simulink model "untitled"  (R2017a)
settings: Solver=FixedStepAuto  StartTime=0.0  StopTime=inf  RelTol=1e-3
settings Model: Creator=teobaiguera  LastModifiedBy=teobaiguera

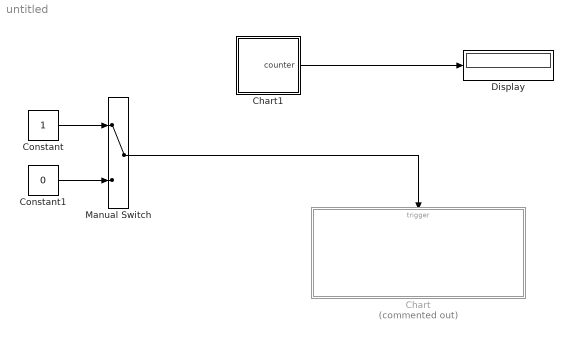
== system untitled ==
  Chart : Stateflow chart  Commented=on  TreatAsAtomicUnit=on
  Chart1 : Stateflow chart  TreatAsAtomicUnit=on
  Constant : Constant
  Constant1 : Constant  Value=0
  Display : Display
  Manual Switch : ManualSwitch
  wires:
  Constant/1 -> Manual Switch/1
  Constant1/1 -> Manual Switch/2
  Manual Switch/1 -> Chart/Trigger
  Chart1/1(counter) -> Display/1

== stateflow chart untitled/Chart1 ==
  state RED
  state GREEN
  state YELLOW
  (default) -> RED
  GREEN -> RED : after(1000,sec)
  RED -> YELLOW : after(1000,sec){counter = counter+1}
  YELLOW -> GREEN : after(1000,sec)
  data: counter output =0

== stateflow chart untitled/Chart ==
  state RED
  state YELLOW
  state GREEN
  YELLOW -> RED : sm_data[after(10,sec)]
  (default) -> RED
  RED -> GREEN : sm_data[after(10,sec)]
  GREEN -> YELLOW : sm_data[after(10,sec)]
  data: counter local double
  events: sm_data input EITHER_EDGE_EVENT
